simulink model "inner_hair_cell"  (R2020b)
settings: Solver=FixedStepDiscrete  StartTime=0.0  StopTime=stopTime  FixedStep=2.0833333333333333e-05  RelTol=1e-3
settings Model: Creator=Ross  LastModifiedBy=conno
settings DataIOCC: SaveOutput=off  SaveTime=off  ReturnWorkspaceOutputs=off
settings OptimizationCC: BlockReduction=off  ConditionallyExecuteInputs=off  DefaultParameterBehavior=Inlined
settings DebuggingCC: ReadBeforeWriteMsg=DisableAll  WriteAfterWriteMsg=DisableAll  WriteAfterReadMsg=DisableAll  AlgebraicLoopMsg=error  MultiTaskDSMMsg=none  SingleTaskRateTransMsg=error  PregeneratedLibrarySubsystemCodeDiagnostic=none  ArithmeticOperatorsInVariantConditions=warning
settings HardwareCC: ProdBitPerPointer=32  ProdBitPerSizeT=32  ProdBitPerPtrDiffT=32  ProdLargestAtomicFloat=None  ProdIntDivRoundTo=Undefined  ProdEndianess=Unspecified  ProdWordSize=32  ProdHWDeviceType=ASIC/FPGA->ASIC/FPGA  TargetBitPerPointer=64  TargetBitPerSizeT=64  TargetBitPerPtrDiffT=64  TargetLongLongMode=on  TargetIntDivRoundTo=Zero  TargetEndianess=LittleEndian  TargetWordSize=64  TargetHWDeviceType=Custom Processor->MATLAB Host Computer  ProdEqTarget=off
settings ModelReferenceCC: UpdateModelReferenceTargets=IfOutOfDate
settings SFSimCC: SFSimEcho=off  SimUseLocalCustomCode=off  CustomCodeUndefinedFunction=UseInterfaceOnly
settings RTWCC: RTWUseLocalCustomCode=off

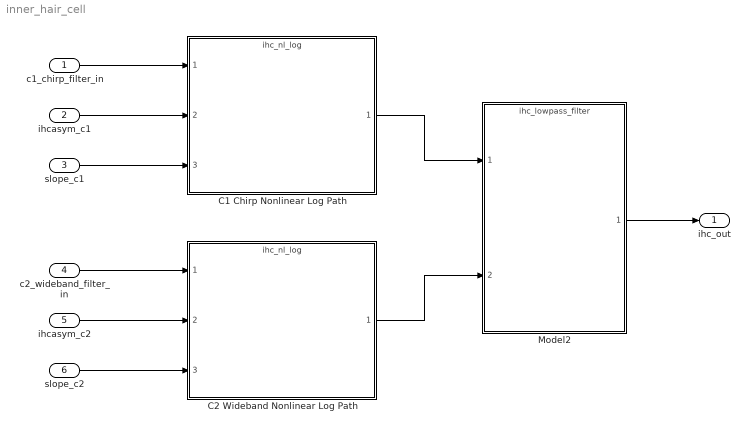
== system inner_hair_cell ==
  c1_chirp_filter_in : Inport  OutDataTypeStr=single  PortDimensions=1  SampleTime=[2.0833333333333333e-05,0]
  ihcasym_c1 : Inport  Port=2  OutDataTypeStr=single  PortDimensions=1  SampleTime=[2.0833333333333333e-05,0]
  slope_c1 : Inport  Port=3  OutDataTypeStr=single  PortDimensions=1  SampleTime=[2.0833333333333333e-05,0]
  c2_wideband_filter_in : Inport  Port=4  OutDataTypeStr=single  PortDimensions=1  SampleTime=[2.0833333333333333e-05,0]
  ihcasym_c2 : Inport  Port=5  OutDataTypeStr=single  PortDimensions=1  SampleTime=[2.0833333333333333e-05,0]
  slope_c2 : Inport  Port=6  OutDataTypeStr=single  PortDimensions=1  SampleTime=[2.0833333333333333e-05,0]
  C1 Chirp Nonlinear Log Path : ModelReference  ModelNameDialog=ihc_nl_log.slx  SimulationMode=Normal  ModelReferenceVersion=1.125
  C2 Wideband Nonlinear Log Path : ModelReference  ModelNameDialog=ihc_nl_log.slx  SimulationMode=Normal  ModelReferenceVersion=1.125
  Model2 : ModelReference  ModelNameDialog=ihc_lowpass_filter.slx  SimulationMode=Normal  ModelReferenceVersion=1.124
  ihc_out : Outport  OutDataTypeStr=single  PortDimensions=1  SampleTime=[2.0833333333333333e-05,0]  InitialOutput=0  VectorParamsAs1DForOutWhenUnconnected=off
  wires:
  C1 Chirp Nonlinear Log Path/1 -> Model2/1
  Model2/1 -> ihc_out/1
  c1_chirp_filter_in/1 -> C1 Chirp Nonlinear Log Path/1
  slope_c1/1 -> C1 Chirp Nonlinear Log Path/3
  slope_c2/1 -> C2 Wideband Nonlinear Log Path/3
  c2_wideband_filter_in/1 -> C2 Wideband Nonlinear Log Path/1
  C2 Wideband Nonlinear Log Path/1 -> Model2/2
  ihcasym_c1/1 -> C1 Chirp Nonlinear Log Path/2
  ihcasym_c2/1 -> C2 Wideband Nonlinear Log Path/2
